simulink model "BaseEngineController_LS"  (Simulink 7.7)
settings: Solver=FixedStepDiscrete  StartTime=0.0  StopTime=10.0  RelTol=1e-3
PreLoadFcn:
  | try, eval([bdroot '_setup']); catch, eval('model_setup', ''); end
InitFcn:
  | try, eval([bdroot '_setup']); catch, eval('model_setup', ''); end
undefined symbols (not defined in the file): ECU555, High, motohawk_build_version, motohawk_trunc_name, motohawk_vardec_config_group, motohawk_vardec_path, True
libraries: MotoHawk_lib x1418, motohawk_control_primitives_lib x183, motohawk_engine_lib x32, simulink x21, motohawk_annotations_lib x9, AutoDoc_lib x8, simulink_extras x4, motohawk_ccp_examples_lib x1, motohawk_control_primitives_motoshare_lib x1
(part 15 of 27)

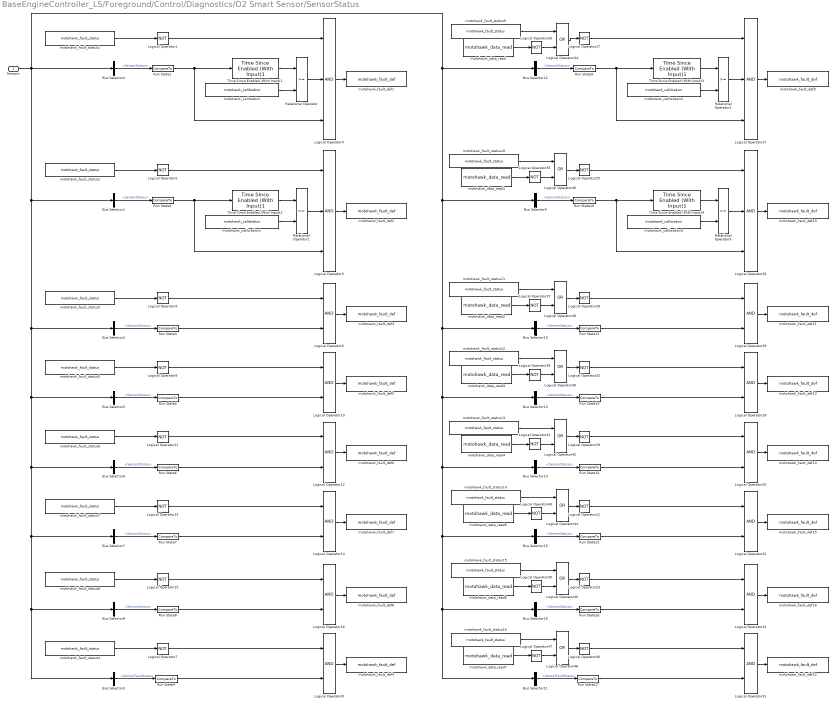
== system BaseEngineController_LS/Foreground/Control/Diagnostics/O2 Smart Sensor/SensorStatus ==
  Sensors : Inport
  Bus Selector{1..2,4..8} (7 alike) : BusSelector  OutputSignals=Raw.CAN.O2_BUS.BANK1.SensorStatus
  Bus Selector{9..10,12..16} (7 alike) : BusSelector  OutputSignals=Raw.CAN.O2_BUS.BANK2.SensorStatus
  Bus Selector11 : BusSelector  OutputSignals=Raw.CAN.O2_BUS.BANK2.SensorFaultState
  Bus Selector3 : BusSelector  OutputSignals=Raw.CAN.O2_BUS.BANK1.SensorFaultState
  Logical Operator{1..2,5,7,9,11,13,15,17,19,21,23,25,28,30,32..33,35,37,39,41,43,45,47} (24 alike) : Logic  Operator=NOT  Inputs=3  AllPortsSameDT=off  OutDataTypeStr=boolean
  Logical Operator{6,8,10,12,14,16,18,20,22,24,29,31} (12 alike) : Logic  AllPortsSameDT=off  OutDataTypeStr=boolean
  Logical Operator{3..4,26..27} (4 alike) : Logic  Inputs=3  AllPortsSameDT=off  OutDataTypeStr=boolean
  Logical Operator{34,36,38,40,42,44,46,48} (8 alike) : Logic  Operator=OR  AllPortsSameDT=off  OutDataTypeStr=boolean
  Relational Operator{,1..3} (4 alike) : RelationalOperator  OutDataTypeStr=boolean
  Run State1 : motohawk_control_primitives_lib/CompareTo  SystemSampleTime=-1  op===  val=0
  Run State{2,4,10,12} (4 alike) : motohawk_control_primitives_lib/CompareTo  SystemSampleTime=-1  op===  val=1
  Run State11 : motohawk_control_primitives_lib/CompareTo  SystemSampleTime=-1  op===  val=7
  Run State13 : motohawk_control_primitives_lib/CompareTo  SystemSampleTime=-1  op===  val=8
  Run State14 : motohawk_control_primitives_lib/CompareTo  SystemSampleTime=-1  op===  val=9
  Run State15 : motohawk_control_primitives_lib/CompareTo  SystemSampleTime=-1  op===  val=10
  Run State16 : motohawk_control_primitives_lib/CompareTo  SystemSampleTime=-1  op===  val=20
  Run State3 : motohawk_control_primitives_lib/CompareTo  SystemSampleTime=-1  op===  val=7
  Run State5 : motohawk_control_primitives_lib/CompareTo  SystemSampleTime=-1  op===  val=8
  Run State6 : motohawk_control_primitives_lib/CompareTo  SystemSampleTime=-1  op===  val=9
  Run State7 : motohawk_control_primitives_lib/CompareTo  SystemSampleTime=-1  op===  val=10
  Run State8 : motohawk_control_primitives_lib/CompareTo  SystemSampleTime=-1  op===  val=20
  Run State9 : motohawk_control_primitives_lib/CompareTo  SystemSampleTime=-1  op===  val=0
  Time Since Enabled (With Input)1 : motohawk_control_primitives_lib/Time Since Enabled (With Input)1  SystemSampleTime=-1  nam='Lam1ResetTime'  samp_time=-1  init=0  upperlim=16000
  Time Since Enabled (With Input)2 : motohawk_control_primitives_lib/Time Since Enabled (With Input)1  SystemSampleTime=-1  nam='Lam1WarmupTime'  samp_time=-1  init=0  upperlim=16000
  Time Since Enabled (With Input)3 : motohawk_control_primitives_lib/Time Since Enabled (With Input)1  SystemSampleTime=-1  nam='Lam2ResetTime'  samp_time=-1  init=0  upperlim=16000
  Time Since Enabled (With Input)4 : motohawk_control_primitives_lib/Time Since Enabled (With Input)1  SystemSampleTime=-1  nam='Lam2WarmupTime'  samp_time=-1  init=0  upperlim=16000
  motohawk_calibration : MotoHawk_lib/Calibration & Probing Blocks/motohawk_calibration  nam='O2Diag_Lam1_StuckInResetThresh'  val=30  storage=Calibration  show_more=off  name_source=Use Parameter  data_type=Inherit from 'Default Value'  read_level=1  write_level=1  ovr_cals=on  view_as=Number  enum_struct={'Disabled', 'Enabled'}  vector_style=Wide Row  use_help_units=off  help=''  units=''  use_header_enum=off  row_header_enum={}  col_header_enum={}  use_min_max=off  min_val=-inf  max_val=inf  use_precision=off  precision=''  gain=1  offset=0  exp=1  use_mototune_group=off  mototune_group=motohawk_vardec_path(gcb)
  motohawk_calibration1 : MotoHawk_lib/Calibration & Probing Blocks/motohawk_calibration  nam='O2Diag_Lam1_StuckInWarmup'  val=30  storage=Calibration  show_more=off  name_source=Use Parameter  data_type=Inherit from 'Default Value'  read_level=1  write_level=1  ovr_cals=on  view_as=Number  enum_struct={'Disabled', 'Enabled'}  vector_style=Wide Row  use_help_units=off  help=''  units=''  use_header_enum=off  row_header_enum={}  col_header_enum={}  use_min_max=off  min_val=-inf  max_val=inf  use_precision=off  precision=''  gain=1  offset=0  exp=1  use_mototune_group=off  mototune_group=motohawk_vardec_path(gcb)
  motohawk_calibration2 : MotoHawk_lib/Calibration & Probing Blocks/motohawk_calibration  nam='O2Diag_Lam21_StuckInResetThresh'  val=30  storage=Calibration  show_more=off  name_source=Use Parameter  data_type=Inherit from 'Default Value'  read_level=1  write_level=1  ovr_cals=on  view_as=Number  enum_struct={'Disabled', 'Enabled'}  vector_style=Wide Row  use_help_units=off  help=''  units=''  use_header_enum=off  row_header_enum={}  col_header_enum={}  use_min_max=off  min_val=-inf  max_val=inf  use_precision=off  precision=''  gain=1  offset=0  exp=1  use_mototune_group=off  mototune_group=motohawk_vardec_path(gcb)
  motohawk_calibration3 : MotoHawk_lib/Calibration & Probing Blocks/motohawk_calibration  nam='O2Diag_Lam2_StuckInWarmup'  val=30  storage=Calibration  show_more=off  name_source=Use Parameter  data_type=Inherit from 'Default Value'  read_level=1  write_level=1  ovr_cals=on  view_as=Number  enum_struct={'Disabled', 'Enabled'}  vector_style=Wide Row  use_help_units=off  help=''  units=''  use_header_enum=off  row_header_enum={}  col_header_enum={}  use_min_max=off  min_val=-inf  max_val=inf  use_precision=off  precision=''  gain=1  offset=0  exp=1  use_mototune_group=off  mototune_group=motohawk_vardec_path(gcb)
  motohawk_data_read{,1..7} (8 alike) : MotoHawk_lib/Data Storage Blocks/motohawk_data_read  source=Lookup By Name  structure=Scalar  operation=Read scalar from location by index  sz_vec=4  sz_row=2  sz_col=3  typ=boolean  nam='BankB_Enbl'  checkNull=on  struct_inst_name='MyData'  struct_nam='MyStruct'
  motohawk_fault_def1 : MotoHawk_lib/Fault Management Blocks/motohawk_fault_def  nam='Lambda1StuckInReset_Fault'  mode=Enabled  id=[]  x=25  y=50  input_suspected=on  indeterminate=off  increment_xy=on  downsample_count=1  ovr_cals=on  ovr_actions=on  show_actions=on  action1_name=''  action1_cond=(None)  action2_name=''  action2_cond=(None)  action3_name=''  action3_cond=(None)  action4_name=''  action4_cond=(None)
  motohawk_fault_def10 : MotoHawk_lib/Fault Management Blocks/motohawk_fault_def  nam='Lambda2StuckInWarmup_Fault'  mode=Enabled  id=[]  x=25  y=50  input_suspected=on  indeterminate=off  increment_xy=on  downsample_count=1  ovr_cals=on  ovr_actions=on  show_actions=on  action1_name=''  action1_cond=(None)  action2_name=''  action2_cond=(None)  action3_name=''  action3_cond=(None)  action4_name=''  action4_cond=(None)
  motohawk_fault_def11 : MotoHawk_lib/Fault Management Blocks/motohawk_fault_def  nam='Lambda2Overheat_Fault'  mode=Enabled  id=[]  x=25  y=50  input_suspected=on  indeterminate=off  increment_xy=on  downsample_count=1  ovr_cals=on  ovr_actions=on  show_actions=on  action1_name=''  action1_cond=(None)  action2_name=''  action2_cond=(None)  action3_name=''  action3_cond=(None)  action4_name=''  action4_cond=(None)
  motohawk_fault_def12 : MotoHawk_lib/Fault Management Blocks/motohawk_fault_def  nam='Lambda2Fault_Fault'  mode=Enabled  id=[]  x=25  y=50  input_suspected=on  indeterminate=off  increment_xy=on  downsample_count=1  ovr_cals=on  ovr_actions=on  show_actions=on  action1_name=''  action1_cond=(None)  action2_name=''  action2_cond=(None)  action3_name=''  action3_cond=(None)  action4_name=''  action4_cond=(None)
  motohawk_fault_def13 : MotoHawk_lib/Fault Management Blocks/motohawk_fault_def  nam='Lambda2Overcool_Fault'  mode=Enabled  id=[]  x=25  y=50  input_suspected=on  indeterminate=off  increment_xy=on  downsample_count=1  ovr_cals=on  ovr_actions=on  show_actions=on  action1_name=''  action1_cond=(None)  action2_name=''  action2_cond=(None)  action3_name=''  action3_cond=(None)  action4_name=''  action4_cond=(None)
  motohawk_fault_def14 : MotoHawk_lib/Fault Management Blocks/motohawk_fault_def  nam='Lambda2HtrShort_Fault'  mode=Enabled  id=[]  x=25  y=50  input_suspected=on  indeterminate=off  increment_xy=on  downsample_count=1  ovr_cals=on  ovr_actions=on  show_actions=on  action1_name=''  action1_cond=(None)  action2_name=''  action2_cond=(None)  action3_name=''  action3_cond=(None)  action4_name=''  action4_cond=(None)
  motohawk_fault_def15 : MotoHawk_lib/Fault Management Blocks/motohawk_fault_def  nam='Lambda2HtrOpen_Fault'  mode=Enabled  id=[]  x=25  y=50  input_suspected=on  indeterminate=off  increment_xy=on  downsample_count=1  ovr_cals=on  ovr_actions=on  show_actions=on  action1_name=''  action1_cond=(None)  action2_name=''  action2_cond=(None)  action3_name=''  action3_cond=(None)  action4_name=''  action4_cond=(None)
  motohawk_fault_def16 : MotoHawk_lib/Fault Management Blocks/motohawk_fault_def  nam='Lambda2Error_Fault'  mode=Enabled  id=[]  x=25  y=50  input_suspected=on  indeterminate=off  increment_xy=on  downsample_count=1  ovr_cals=on  ovr_actions=on  show_actions=on  action1_name=''  action1_cond=(None)  action2_name=''  action2_cond=(None)  action3_name=''  action3_cond=(None)  action4_name=''  action4_cond=(None)
  motohawk_fault_def2 : MotoHawk_lib/Fault Management Blocks/motohawk_fault_def  nam='Lambda1StuckInWarmup_Fault'  mode=Enabled  id=[]  x=25  y=50  input_suspected=on  indeterminate=off  increment_xy=on  downsample_count=1  ovr_cals=on  ovr_actions=on  show_actions=on  action1_name=''  action1_cond=(None)  action2_name=''  action2_cond=(None)  action3_name=''  action3_cond=(None)  action4_name=''  action4_cond=(None)
  motohawk_fault_def3 : MotoHawk_lib/Fault Management Blocks/motohawk_fault_def  nam='Lambda1Overheat_Fault'  mode=Enabled  id=[]  x=25  y=50  input_suspected=on  indeterminate=off  increment_xy=on  downsample_count=1  ovr_cals=on  ovr_actions=on  show_actions=on  action1_name=''  action1_cond=(None)  action2_name=''  action2_cond=(None)  action3_name=''  action3_cond=(None)  action4_name=''  action4_cond=(None)
  motohawk_fault_def4 : MotoHawk_lib/Fault Management Blocks/motohawk_fault_def  nam='Lambda1Fault_Fault'  mode=Enabled  id=[]  x=25  y=50  input_suspected=on  indeterminate=off  increment_xy=on  downsample_count=1  ovr_cals=on  ovr_actions=on  show_actions=on  action1_name=''  action1_cond=(None)  action2_name=''  action2_cond=(None)  action3_name=''  action3_cond=(None)  action4_name=''  action4_cond=(None)
  motohawk_fault_def5 : MotoHawk_lib/Fault Management Blocks/motohawk_fault_def  nam='Lambda1Overcool_Fault'  mode=Enabled  id=[]  x=25  y=50  input_suspected=on  indeterminate=off  increment_xy=on  downsample_count=1  ovr_cals=on  ovr_actions=on  show_actions=on  action1_name=''  action1_cond=(None)  action2_name=''  action2_cond=(None)  action3_name=''  action3_cond=(None)  action4_name=''  action4_cond=(None)
  motohawk_fault_def6 : MotoHawk_lib/Fault Management Blocks/motohawk_fault_def  nam='Lambda1HtrShort_Fault'  mode=Enabled  id=[]  x=25  y=50  input_suspected=on  indeterminate=off  increment_xy=on  downsample_count=1  ovr_cals=on  ovr_actions=on  show_actions=on  action1_name=''  action1_cond=(None)  action2_name=''  action2_cond=(None)  action3_name=''  action3_cond=(None)  action4_name=''  action4_cond=(None)
  motohawk_fault_def7 : MotoHawk_lib/Fault Management Blocks/motohawk_fault_def  nam='Lambda1HtrOpen_Fault'  mode=Enabled  id=[]  x=25  y=50  input_suspected=on  indeterminate=off  increment_xy=on  downsample_count=1  ovr_cals=on  ovr_actions=on  show_actions=on  action1_name=''  action1_cond=(None)  action2_name=''  action2_cond=(None)  action3_name=''  action3_cond=(None)  action4_name=''  action4_cond=(None)
  motohawk_fault_def8 : MotoHawk_lib/Fault Management Blocks/motohawk_fault_def  nam='Lambda1Error_Fault'  mode=Enabled  id=[]  x=25  y=50  input_suspected=on  indeterminate=off  increment_xy=on  downsample_count=1  ovr_cals=on  ovr_actions=on  show_actions=on  action1_name=''  action1_cond=(None)  action2_name=''  action2_cond=(None)  action3_name=''  action3_cond=(None)  action4_name=''  action4_cond=(None)
  motohawk_fault_def9 : MotoHawk_lib/Fault Management Blocks/motohawk_fault_def  nam='Lambda2StuckInReset_Fault'  mode=Enabled  id=[]  x=25  y=50  input_suspected=on  indeterminate=off  increment_xy=on  downsample_count=1  ovr_cals=on  ovr_actions=on  show_actions=on  action1_name=''  action1_cond=(None)  action2_name=''  action2_cond=(None)  action3_name=''  action3_cond=(None)  action4_name=''  action4_cond=(None)
  motohawk_fault_status{1..8} (8 alike) : MotoHawk_lib/Fault Management Blocks/motohawk_fault_status  source=Lookup By Name  nam='Lambda_1_Timeout'  status=Active
  motohawk_fault_status{9..16} (8 alike) : MotoHawk_lib/Fault Management Blocks/motohawk_fault_status  source=Lookup By Name  nam='Lambda_2_Timeout'  status=Active
  wires:
  Logical Operator4/1 -> motohawk_fault_def1/1
  motohawk_fault_status1/1 -> Logical Operator1/1
  Sensors/1 -> Bus Selector4/1, Bus Selector1/1, Bus Selector2/1, Bus Selector5/1, Bus Selector6/1, Bus Selector7/1, Bus Selector8/1, Bus Selector3/1, Bus Selector12/1, Bus Selector9/1, Bus Selector10/1, Bus Selector13/1, Bus Selector14/1, Bus Selector15/1, Bus Selector11/1, Bus Selector16/1
  Logical Operator1/1 -> Logical Operator4/1
  Bus Selector4/1 -> Run State1/1  "<SensorStatus>"
  Time Since Enabled (With Input)1/1 -> Relational Operator/1
  motohawk_calibration/1 -> Relational Operator/2
  Run State1/1 -> Time Since Enabled (With Input)1/1, Logical Operator4/3
  Relational Operator/1 -> Logical Operator4/2
  Logical Operator3/1 -> motohawk_fault_def2/1
  motohawk_fault_status2/1 -> Logical Operator2/1
  Logical Operator2/1 -> Logical Operator3/1
  Bus Selector1/1 -> Run State2/1  "<SensorStatus>"
  Time Since Enabled (With Input)2/1 -> Relational Operator1/1
  motohawk_calibration1/1 -> Relational Operator1/2
  Run State2/1 -> Time Since Enabled (With Input)2/1, Logical Operator3/3
  Relational Operator1/1 -> Logical Operator3/2
  Logical Operator6/1 -> motohawk_fault_def3/1
  motohawk_fault_status3/1 -> Logical Operator5/1
  Logical Operator5/1 -> Logical Operator6/1
  Bus Selector2/1 -> Run State3/1  "<SensorStatus>"
  Run State3/1 -> Logical Operator6/2
  Logical Operator8/1 -> motohawk_fault_def4/1
  motohawk_fault_status4/1 -> Logical Operator7/1
  Logical Operator7/1 -> Logical Operator8/1
  Bus Selector3/1 -> Run State4/1  "<SensorFaultState>"
  Run State4/1 -> Logical Operator8/2
  Logical Operator10/1 -> motohawk_fault_def5/1
  motohawk_fault_status5/1 -> Logical Operator9/1
  Logical Operator9/1 -> Logical Operator10/1
  Bus Selector5/1 -> Run State5/1  "<SensorStatus>"
  Run State5/1 -> Logical Operator10/2
  Logical Operator12/1 -> motohawk_fault_def6/1
  motohawk_fault_status6/1 -> Logical Operator11/1
  Logical Operator11/1 -> Logical Operator12/1
  Bus Selector6/1 -> Run State6/1  "<SensorStatus>"
  Run State6/1 -> Logical Operator12/2
  Logical Operator14/1 -> motohawk_fault_def7/1
  motohawk_fault_status7/1 -> Logical Operator13/1
  Logical Operator13/1 -> Logical Operator14/1
  Bus Selector7/1 -> Run State7/1  "<SensorStatus>"
  Run State7/1 -> Logical Operator14/2
  Logical Operator16/1 -> motohawk_fault_def8/1
  motohawk_fault_status8/1 -> Logical Operator15/1
  Logical Operator15/1 -> Logical Operator16/1
  Bus Selector8/1 -> Run State8/1  "<SensorStatus>"
  Run State8/1 -> Logical Operator16/2
  Logical Operator27/1 -> motohawk_fault_def9/1
  Logical Operator17/1 -> Logical Operator27/1
  Bus Selector12/1 -> Run State9/1  "<SensorStatus>"
  Time Since Enabled (With Input)3/1 -> Relational Operator2/1
  motohawk_calibration2/1 -> Relational Operator2/2
  Run State9/1 -> Time Since Enabled (With Input)3/1, Logical Operator27/3
  Relational Operator2/1 -> Logical Operator27/2
  Logical Operator26/1 -> motohawk_fault_def10/1
  Logical Operator25/1 -> Logical Operator26/1
  Bus Selector9/1 -> Run State10/1  "<SensorStatus>"
  Time Since Enabled (With Input)4/1 -> Relational Operator3/1
  motohawk_calibration3/1 -> Relational Operator3/2
  Run State10/1 -> Time Since Enabled (With Input)4/1, Logical Operator26/3
  Relational Operator3/1 -> Logical Operator26/2
  Logical Operator29/1 -> motohawk_fault_def11/1
  Logical Operator28/1 -> Logical Operator29/1
  Bus Selector10/1 -> Run State11/1  "<SensorStatus>"
  Run State11/1 -> Logical Operator29/2
  Logical Operator31/1 -> motohawk_fault_def12/1
  Logical Operator30/1 -> Logical Operator31/1
  Bus Selector11/1 -> Run State12/1  "<SensorFaultState>"
  Run State12/1 -> Logical Operator31/2
  Logical Operator18/1 -> motohawk_fault_def13/1
  Logical Operator32/1 -> Logical Operator18/1
  Bus Selector13/1 -> Run State13/1  "<SensorStatus>"
  Run State13/1 -> Logical Operator18/2
  Logical Operator20/1 -> motohawk_fault_def14/1
  Logical Operator19/1 -> Logical Operator20/1
  Bus Selector14/1 -> Run State14/1  "<SensorStatus>"
  Run State14/1 -> Logical Operator20/2
  Logical Operator22/1 -> motohawk_fault_def15/1
  Logical Operator21/1 -> Logical Operator22/1
  Bus Selector15/1 -> Run State15/1  "<SensorStatus>"
  Run State15/1 -> Logical Operator22/2
  Logical Operator24/1 -> motohawk_fault_def16/1
  Logical Operator23/1 -> Logical Operator24/1
  Bus Selector16/1 -> Run State16/1  "<SensorStatus>"
  Run State16/1 -> Logical Operator24/2
  motohawk_data_read/1 -> Logical Operator33/1
  Logical Operator33/1 -> Logical Operator34/2
  motohawk_fault_status9/1 -> Logical Operator34/1
  Logical Operator34/1 -> Logical Operator17/1
  motohawk_data_read1/1 -> Logical Operator35/1
  Logical Operator35/1 -> Logical Operator36/2
  motohawk_fault_status10/1 -> Logical Operator36/1
  Logical Operator36/1 -> Logical Operator25/1
  motohawk_data_read2/1 -> Logical Operator37/1
  Logical Operator37/1 -> Logical Operator38/2
  motohawk_fault_status11/1 -> Logical Operator38/1
  Logical Operator38/1 -> Logical Operator28/1
  motohawk_data_read3/1 -> Logical Operator39/1
  Logical Operator39/1 -> Logical Operator40/2
  motohawk_fault_status12/1 -> Logical Operator40/1
  Logical Operator40/1 -> Logical Operator32/1
  motohawk_data_read4/1 -> Logical Operator41/1
  Logical Operator41/1 -> Logical Operator42/2
  motohawk_fault_status13/1 -> Logical Operator42/1
  Logical Operator42/1 -> Logical Operator19/1
  motohawk_data_read5/1 -> Logical Operator43/1
  Logical Operator43/1 -> Logical Operator44/2
  motohawk_fault_status14/1 -> Logical Operator44/1
  Logical Operator44/1 -> Logical Operator21/1
  motohawk_data_read6/1 -> Logical Operator45/1
  Logical Operator45/1 -> Logical Operator46/2
  motohawk_fault_status15/1 -> Logical Operator46/1
  Logical Operator46/1 -> Logical Operator23/1
  motohawk_data_read7/1 -> Logical Operator47/1
  Logical Operator47/1 -> Logical Operator48/2
  motohawk_fault_status16/1 -> Logical Operator48/1
  Logical Operator48/1 -> Logical Operator30/1

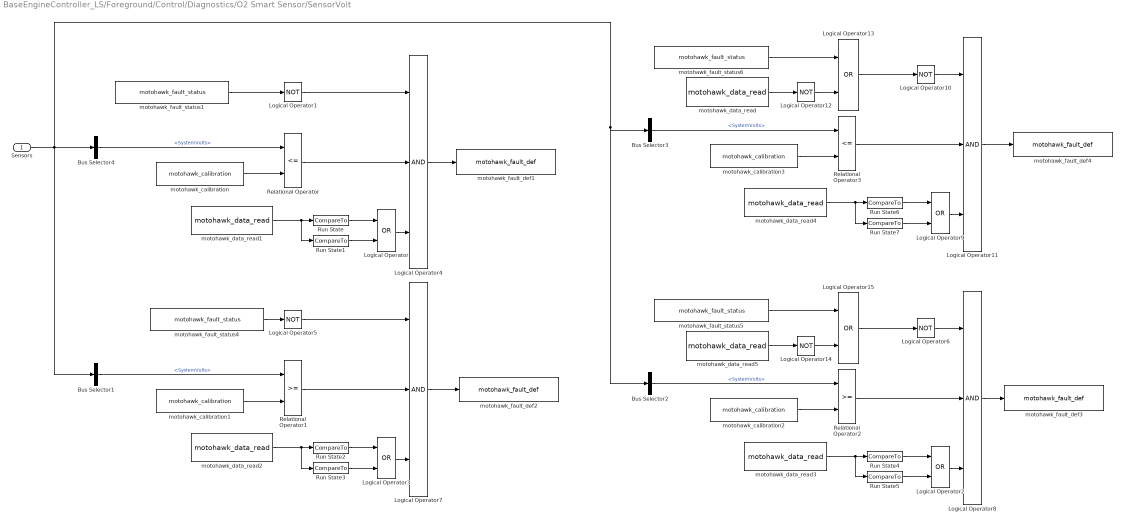
== system BaseEngineController_LS/Foreground/Control/Diagnostics/O2 Smart Sensor/SensorVolt ==
  Sensors : Inport
  Bus Selector1 : BusSelector  OutputSignals=Raw.CAN.O2_BUS.BANK1.SystemVolts
  Bus Selector2 : BusSelector  OutputSignals=Raw.CAN.O2_BUS.BANK2.SystemVolts
  Bus Selector3 : BusSelector  OutputSignals=Raw.CAN.O2_BUS.BANK2.SystemVolts
  Bus Selector4 : BusSelector  OutputSignals=Raw.CAN.O2_BUS.BANK1.SystemVolts
  Logical Operator{,2..3,9,13,15} (6 alike) : Logic  Operator=OR  AllPortsSameDT=off  OutDataTypeStr=boolean
  Logical Operator{1,5..6,10,12,14} (6 alike) : Logic  Operator=NOT  Inputs=3  AllPortsSameDT=off  OutDataTypeStr=boolean
  Logical Operator{4,7..8,11} (4 alike) : Logic  Inputs=3  AllPortsSameDT=off  OutDataTypeStr=boolean
  Relational Operator : RelationalOperator  Operator=<=  OutDataTypeStr=boolean
  Relational Operator1 : RelationalOperator  OutDataTypeStr=boolean
  Relational Operator2 : RelationalOperator  OutDataTypeStr=boolean
  Relational Operator3 : RelationalOperator  Operator=<=  OutDataTypeStr=boolean
  Run State{,2,4,6} (4 alike) : motohawk_control_primitives_lib/CompareTo  SystemSampleTime=-1  op===  val=3
  Run State{1,3,5,7} (4 alike) : motohawk_control_primitives_lib/CompareTo  SystemSampleTime=-1  op===  val=2
  motohawk_calibration : MotoHawk_lib/Calibration & Probing Blocks/motohawk_calibration  nam='Lambda1_VoltLowThresh'  val=10  storage=Calibration  show_more=off  name_source=Use Parameter  data_type=Inherit from 'Default Value'  read_level=1  write_level=1  ovr_cals=on  view_as=Number  enum_struct={'Disabled', 'Enabled'}  vector_style=Wide Row  use_help_units=off  help=''  units=''  use_header_enum=off  row_header_enum={}  col_header_enum={}  use_min_max=off  min_val=-inf  max_val=inf  use_precision=off  precision=''  gain=1  offset=0  exp=1  use_mototune_group=off  mototune_group=motohawk_vardec_path(gcb)
  motohawk_calibration1 : MotoHawk_lib/Calibration & Probing Blocks/motohawk_calibration  nam='Lambda1_VoltHighThresh'  val=15  storage=Calibration  show_more=off  name_source=Use Parameter  data_type=Inherit from 'Default Value'  read_level=1  write_level=1  ovr_cals=on  view_as=Number  enum_struct={'Disabled', 'Enabled'}  vector_style=Wide Row  use_help_units=off  help=''  units=''  use_header_enum=off  row_header_enum={}  col_header_enum={}  use_min_max=off  min_val=-inf  max_val=inf  use_precision=off  precision=''  gain=1  offset=0  exp=1  use_mototune_group=off  mototune_group=motohawk_vardec_path(gcb)
  motohawk_calibration2 : MotoHawk_lib/Calibration & Probing Blocks/motohawk_calibration  nam='Lambda2_VoltHighThresh'  val=15  storage=Calibration  show_more=off  name_source=Use Parameter  data_type=Inherit from 'Default Value'  read_level=1  write_level=1  ovr_cals=on  view_as=Number  enum_struct={'Disabled', 'Enabled'}  vector_style=Wide Row  use_help_units=off  help=''  units=''  use_header_enum=off  row_header_enum={}  col_header_enum={}  use_min_max=off  min_val=-inf  max_val=inf  use_precision=off  precision=''  gain=1  offset=0  exp=1  use_mototune_group=off  mototune_group=motohawk_vardec_path(gcb)
  motohawk_calibration3 : MotoHawk_lib/Calibration & Probing Blocks/motohawk_calibration  nam='Lambda2_VoltLowThresh'  val=10  storage=Calibration  show_more=off  name_source=Use Parameter  data_type=Inherit from 'Default Value'  read_level=1  write_level=1  ovr_cals=on  view_as=Number  enum_struct={'Disabled', 'Enabled'}  vector_style=Wide Row  use_help_units=off  help=''  units=''  use_header_enum=off  row_header_enum={}  col_header_enum={}  use_min_max=off  min_val=-inf  max_val=inf  use_precision=off  precision=''  gain=1  offset=0  exp=1  use_mototune_group=off  mototune_group=motohawk_vardec_path(gcb)
  motohawk_data_read : MotoHawk_lib/Data Storage Blocks/motohawk_data_read  source=Lookup By Name  structure=Scalar  operation=Read scalar from location by index  sz_vec=4  sz_row=2  sz_col=3  typ=boolean  nam='BankB_Enbl'  checkNull=on  struct_inst_name='MyData'  struct_nam='MyStruct'
  motohawk_data_read{1..4} (4 alike) : MotoHawk_lib/Data Storage Blocks/motohawk_data_read  source=Lookup By Name  structure=Scalar  operation=Read entire data structure at once  sz_vec=4  sz_row=2  sz_col=3  typ=uint8  nam='EngineState'  checkNull=on  struct_inst_name='Struct1'  struct_nam='MyStruct'
  motohawk_data_read5 : MotoHawk_lib/Data Storage Blocks/motohawk_data_read  source=Lookup By Name  structure=Scalar  operation=Read scalar from location by index  sz_vec=4  sz_row=2  sz_col=3  typ=boolean  nam='BankB_Enbl'  checkNull=on  struct_inst_name='MyData'  struct_nam='MyStruct'
  motohawk_fault_def1 : MotoHawk_lib/Fault Management Blocks/motohawk_fault_def  nam='Lambda1VoltLow_Fault'  mode=Enabled  id=[]  x=25  y=50  input_suspected=on  indeterminate=off  increment_xy=on  downsample_count=1  ovr_cals=on  ovr_actions=on  show_actions=on  action1_name=''  action1_cond=(None)  action2_name=''  action2_cond=(None)  action3_name=''  action3_cond=(None)  action4_name=''  action4_cond=(None)
  motohawk_fault_def2 : MotoHawk_lib/Fault Management Blocks/motohawk_fault_def  nam='Lambda1VoltHigh_Fault'  mode=Enabled  id=[]  x=25  y=50  input_suspected=on  indeterminate=off  increment_xy=on  downsample_count=1  ovr_cals=on  ovr_actions=on  show_actions=on  action1_name=''  action1_cond=(None)  action2_name=''  action2_cond=(None)  action3_name=''  action3_cond=(None)  action4_name=''  action4_cond=(None)
  motohawk_fault_def3 : MotoHawk_lib/Fault Management Blocks/motohawk_fault_def  nam='Lambda2VoltHigh_Fault'  mode=Enabled  id=[]  x=25  y=50  input_suspected=on  indeterminate=off  increment_xy=on  downsample_count=1  ovr_cals=on  ovr_actions=on  show_actions=on  action1_name=''  action1_cond=(None)  action2_name=''  action2_cond=(None)  action3_name=''  action3_cond=(None)  action4_name=''  action4_cond=(None)
  motohawk_fault_def4 : MotoHawk_lib/Fault Management Blocks/motohawk_fault_def  nam='Lambda2VoltLow_Fault'  mode=Enabled  id=[]  x=25  y=50  input_suspected=on  indeterminate=off  increment_xy=on  downsample_count=1  ovr_cals=on  ovr_actions=on  show_actions=on  action1_name=''  action1_cond=(None)  action2_name=''  action2_cond=(None)  action3_name=''  action3_cond=(None)  action4_name=''  action4_cond=(None)
  motohawk_fault_status1 : MotoHawk_lib/Fault Management Blocks/motohawk_fault_status  source=Lookup By Name  nam='Lambda_1_Timeout'  status=Active
  motohawk_fault_status4 : MotoHawk_lib/Fault Management Blocks/motohawk_fault_status  source=Lookup By Name  nam='Lambda_1_Timeout'  status=Active
  motohawk_fault_status5 : MotoHawk_lib/Fault Management Blocks/motohawk_fault_status  source=Lookup By Name  nam='Lambda_2_Timeout'  status=Active
  motohawk_fault_status6 : MotoHawk_lib/Fault Management Blocks/motohawk_fault_status  source=Lookup By Name  nam='Lambda_2_Timeout'  status=Active
  wires:
  Sensors/1 -> Bus Selector4/1, Bus Selector1/1, Bus Selector2/1, Bus Selector3/1
  Logical Operator4/1 -> motohawk_fault_def1/1
  Logical Operator1/1 -> Logical Operator4/1
  motohawk_data_read1/1 -> Run State/1, Run State1/1
  Run State1/1 -> Logical Operator/2
  Run State/1 -> Logical Operator/1
  Logical Operator/1 -> Logical Operator4/3
  Bus Selector4/1 -> Relational Operator/1  "<SystemVolts>"
  Relational Operator/1 -> Logical Operator4/2
  motohawk_calibration/1 -> Relational Operator/2
  motohawk_fault_status1/1 -> Logical Operator1/1
  Logical Operator7/1 -> motohawk_fault_def2/1
  Logical Operator5/1 -> Logical Operator7/1
  motohawk_data_read2/1 -> Run State2/1, Run State3/1
  Run State3/1 -> Logical Operator3/2
  Run State2/1 -> Logical Operator3/1
  Logical Operator3/1 -> Logical Operator7/3
  Bus Selector1/1 -> Relational Operator1/1  "<SystemVolts>"
  Relational Operator1/1 -> Logical Operator7/2
  motohawk_calibration1/1 -> Relational Operator1/2
  motohawk_fault_status4/1 -> Logical Operator5/1
  Logical Operator8/1 -> motohawk_fault_def3/1
  motohawk_data_read3/1 -> Run State4/1, Run State5/1
  Run State5/1 -> Logical Operator2/2
  Run State4/1 -> Logical Operator2/1
  Logical Operator2/1 -> Logical Operator8/3
  Bus Selector2/1 -> Relational Operator2/1  "<SystemVolts>"
  Relational Operator2/1 -> Logical Operator8/2
  motohawk_calibration2/1 -> Relational Operator2/2
  Logical Operator11/1 -> motohawk_fault_def4/1
  Logical Operator10/1 -> Logical Operator11/1
  motohawk_data_read4/1 -> Run State6/1, Run State7/1
  Run State7/1 -> Logical Operator9/2
  Run State6/1 -> Logical Operator9/1
  Logical Operator9/1 -> Logical Operator11/3
  Bus Selector3/1 -> Relational Operator3/1  "<SystemVolts>"
  Relational Operator3/1 -> Logical Operator11/2
  motohawk_calibration3/1 -> Relational Operator3/2
  motohawk_data_read/1 -> Logical Operator12/1
  Logical Operator12/1 -> Logical Operator13/2
  motohawk_fault_status6/1 -> Logical Operator13/1
  Logical Operator13/1 -> Logical Operator10/1
  motohawk_data_read5/1 -> Logical Operator14/1
  Logical Operator14/1 -> Logical Operator15/2
  motohawk_fault_status5/1 -> Logical Operator15/1
  Logical Operator15/1 -> Logical Operator6/1
  Logical Operator6/1 -> Logical Operator8/1

== system BaseEngineController_LS/Foreground/Control/Diagnostics/Overspeed Protection/BaseRevLimit ==
  RPM : Inport
  Hysterisis : motohawk_control_primitives_lib/Hysterisis  SystemSampleTime=-1
  Hysterisis1 : motohawk_control_primitives_lib/Hysterisis  SystemSampleTime=-1
  Hysterisis2 : motohawk_control_primitives_lib/Hysterisis  SystemSampleTime=-1
  Logical Operator3 : Logic
  Logical Operator4 : Logic  Operator=NOT
  Logical Operator5 : Logic
  Logical Operator6 : Logic  Operator=NOT
  Overspeed : RelationalOperator  Operator=>  ZeroCross=off  InputSameDT=on
  Overspeed1 : RelationalOperator  Operator=>  ZeroCross=off  InputSameDT=on
  Overspeed2 : RelationalOperator  Operator=>  ZeroCross=off  InputSameDT=on
  Sum1 : Sum  Inputs=+-  SaturateOnIntegerOverflow=on
  Sum2 : Sum  Inputs=+-  SaturateOnIntegerOverflow=on
  Sum3 : Sum  SaturateOnIntegerOverflow=on
  Sum4 : Sum  Inputs=+-  SaturateOnIntegerOverflow=on
  Sum5 : Sum  SaturateOnIntegerOverflow=on
  motohawk_calibration : MotoHawk_lib/Calibration & Probing Blocks/motohawk_calibration  nam='BaseRevLimit'  val=4200  storage=Calibration  show_more=on  name_source=Use Parameter  data_type=int16  read_level=1  write_level=1  ovr_cals=on  view_as=Number  enum_struct={'Disabled', 'Enabled'}  vector_style=Wide Row  use_help_units=on  help='Maximum RPM allowed, before any action is taken'  units='RPM'  use_header_enum=off  row_header_enum={}  col_header_enum={}  use_min_max=on  min_val=0  max_val=inf  use_precision=off  precision=''  gain=1  offset=0  exp=1  use_mototune_group=on  mototune_group=motohawk_vardec_path(gcb)
  motohawk_calibration1 : MotoHawk_lib/Calibration & Probing Blocks/motohawk_calibration  nam='RevLimitHyst'  val=20  storage=Calibration  show_more=on  name_source=Use Parameter  data_type=int16  read_level=1  write_level=1  ovr_cals=on  view_as=Number  enum_struct={'Disabled', 'Enabled'}  vector_style=Wide Row  use_help_units=on  help='Hysteresis applied to MaxRPM once rev limit threshold is satisfied'  units='RPM'  use_header_enum=off  row_header_enum={}  col_header_enum={}  use_min_max=on  min_val=0  max_val=12000  use_precision=off  precision=''  gain=1  offset=0  exp=1  use_mototune_group=on  mototune_group=motohawk_vardec_path(gcb)
  motohawk_calibration2 : MotoHawk_lib/Calibration & Probing Blocks/motohawk_calibration  nam='MediumRevOffset'  val=75  storage=Calibration  show_more=on  name_source=Use Parameter  data_type=int16  read_level=1  write_level=1  ovr_cals=on  view_as=Number  enum_struct={'Disabled', 'Enabled'}  vector_style=Wide Row  use_help_units=on  help='RPM rev limit for medium action to be taken'  units='RPM'  use_header_enum=off  row_header_enum={}  col_header_enum={}  use_min_max=on  min_val=0  max_val=inf  use_precision=off  precision=''  gain=1  offset=0  exp=1  use_mototune_group=on  mototune_group=motohawk_vardec_path(gcb)
  motohawk_calibration4 : MotoHawk_lib/Calibration & Probing Blocks/motohawk_calibration  nam='HardRevOffset'  val=100  storage=Calibration  show_more=on  name_source=Use Parameter  data_type=int16  read_level=1  write_level=1  ovr_cals=on  view_as=Number  enum_struct={'Disabled', 'Enabled'}  vector_style=Wide Row  use_help_units=on  help='RPM rev limit for hard action to be taken'  units='RPM'  use_header_enum=off  row_header_enum={}  col_header_enum={}  use_min_max=on  min_val=0  max_val=inf  use_precision=off  precision=''  gain=1  offset=0  exp=1  use_mototune_group=on  mototune_group=motohawk_vardec_path(gcb)
  Soft : Outport
  Medium : Outport  Port=2
  Hard : Outport  Port=3
  wires:
  Hysterisis2/1 -> Overspeed2/2
  Hysterisis1/1 -> Overspeed1/2
  Hysterisis/1 -> Overspeed/2
  motohawk_calibration1/1 -> Sum2/2, Sum1/2, Sum4/2
  motohawk_calibration/1 -> Sum2/1, Sum3/1, Sum5/1, Hysterisis/1
  RPM/1 -> Overspeed/1, Overspeed1/1, Overspeed2/1, Hysterisis/3, Hysterisis2/3, Hysterisis1/3
  motohawk_calibration2/1 -> Sum3/2
  Sum3/1 -> Sum1/1, Hysterisis1/1
  motohawk_calibration4/1 -> Sum5/2
  Sum5/1 -> Sum4/1, Hysterisis2/1
  Overspeed/1 -> Logical Operator3/1
  Logical Operator3/1 -> Soft/1
  Logical Operator4/1 -> Logical Operator3/2
  Overspeed1/1 -> Logical Operator4/1, Logical Operator5/1
  Logical Operator6/1 -> Logical Operator5/2
  Overspeed2/1 -> Logical Operator6/1, Hard/1
  Logical Operator5/1 -> Medium/1
  Sum2/1 -> Hysterisis/2
  Sum1/1 -> Hysterisis1/2
  Sum4/1 -> Hysterisis2/2

== system BaseEngineController_LS/Foreground/Control/VirtualSensors/AirCalcs/Capture Signal At Startup ==
  note: Count up to "BARO_Count" samples
  Signal_In : Inport
  Enable : EnablePort  StatesWhenEnabling=reset
  Add : Sum
  Add1 : Sum  Inputs=+-
  Collect Average : Subsystem  TreatAsAtomicUnit=on
  Constant : Constant  Value=int8(1)  SampleTime=-1
  Logical Operator : Logic  AllPortsSameDT=off  OutDataTypeStr=boolean
  Relational Operator : RelationalOperator  Operator=<=
  Relational Operator1 : RelationalOperator  Operator=>
  Sum : Sum  Inputs=++|  InputSameDT=on
  Switch : Switch  Threshold=1  ZeroCross=off  InputSameDT=on
  TwoSampleBuffer ToIgnore : Constant  Value=2  OutDataTypeStr=Inherit: Inherit via back propagation  SampleTime=-1
  Unit Delay : UnitDelay  SampleTime=-1
  motohawk_calibration : MotoHawk_lib/Calibration & Probing Blocks/motohawk_calibration  nam='BARO_Count'  val=int8(count)  storage=Calibration  show_more=on  name_source=Use Parameter  data_type=Inherit from 'Default Value'  read_level=1  write_level=1  ovr_cals=on  view_as=Number  enum_struct={'Disabled', 'Enabled'}  vector_style=Wide Row  use_help_units=on  help='Number of samples to average at key-up to produce signal value'  units=''  use_header_enum=off  row_header_enum={}  col_header_enum={}  use_min_max=off  min_val=-inf  max_val=inf  use_precision=off  precision=''  gain=1  offset=0  exp=1  use_mototune_group=on  mototune_group=motohawk_vardec_path(gcb)
  Signal_KeyUp : Outport
  wires:
  Sum/1 -> Switch/1, Relational Operator/1, Relational Operator1/1
  Relational Operator/1 -> Switch/2, Logical Operator/1
  Switch/1 -> Unit Delay/1, Add1/1
  Collect Average/1(Captured_Signal) -> Signal_KeyUp/1
  Signal_In/1 -> Collect Average/2(Signal)
  Unit Delay/1 -> Sum/1
  Constant/1 -> Sum/2
  motohawk_calibration/1 -> Add/1
  Add/1 -> Relational Operator/2, Switch/3
  TwoSampleBuffer ToIgnore/1 -> Add/2, Relational Operator1/2, Add1/2
  Logical Operator/1 -> Collect Average/Enable
  Relational Operator1/1 -> Logical Operator/2
  Add1/1 -> Collect Average/1(Count)

== system BaseEngineController_LS/Foreground/Control/VirtualSensors/AirCalcs/Running Baro Learn ==
  Eng State : Inport
  MAP : Inport  Port=2
  Compare To Constant : simulink/Logic and Bit Operations/Compare To Constant  SystemSampleTime=-1  relop=>  const=1  LogicOutDataTypeMode=uint8
  Data Type Conversion : DataTypeConversion  OutDataTypeStr=boolean
  Logical Operator : Logic  Inputs=3  AllPortsSameDT=off  OutDataTypeStr=boolean
  Product : Product  RndMeth=Zero
  Relational Operator : RelationalOperator  OutDataTypeStr=boolean
  Relational Operator1 : RelationalOperator  OutDataTypeStr=boolean
  Relational Operator2 : RelationalOperator  OutDataTypeStr=boolean
  Time Since Enabled (With Input)1 : motohawk_control_primitives_lib/Time Since Enabled (With Input)1  SystemSampleTime=-1  nam='BaroLearnTmr'  samp_time=-1  init=0  upperlim=16000
  motohawk_calibration : MotoHawk_lib/Calibration & Probing Blocks/motohawk_calibration  nam='BaroLearn_Tm'  val=.2  storage=Calibration  show_more=on  name_source=Use Parameter  data_type=Inherit from 'Default Value'  read_level=1  write_level=1  ovr_cals=on  view_as=Number  enum_struct={'Disabled', 'Enabled'}  vector_style=Wide Row  use_help_units=on  help=''  units='sec'  use_header_enum=off  row_header_enum={}  col_header_enum={}  use_min_max=on  min_val=0  max_val=100  use_precision=off  precision=''  gain=1  offset=0  exp=1  use_mototune_group=off  mototune_group=motohawk_vardec_path(gcb)
  motohawk_calibration1 : MotoHawk_lib/Calibration & Probing Blocks/motohawk_calibration  nam='BaroLearn_TPSPos'  val=95  storage=Calibration  show_more=on  name_source=Use Parameter  data_type=Inherit from 'Default Value'  read_level=1  write_level=1  ovr_cals=on  view_as=Number  enum_struct={'Disabled', 'Enabled'}  vector_style=Wide Row  use_help_units=on  help=''  units='%'  use_header_enum=off  row_header_enum={}  col_header_enum={}  use_min_max=on  min_val=0  max_val=100  use_precision=off  precision=''  gain=1  offset=0  exp=1  use_mototune_group=off  mototune_group=motohawk_vardec_path(gcb)
  motohawk_calibration2 : MotoHawk_lib/Calibration & Probing Blocks/motohawk_calibration  nam='BaroLearn_MAP'  val=95  storage=Calibration  show_more=on  name_source=Use Parameter  data_type=Inherit from 'Default Value'  read_level=1  write_level=1  ovr_cals=on  view_as=Number  enum_struct={'Disabled', 'Enabled'}  vector_style=Wide Row  use_help_units=on  help=''  units='kPa'  use_header_enum=off  row_header_enum={}  col_header_enum={}  use_min_max=on  min_val=0  max_val=100  use_precision=off  precision=''  gain=1  offset=0  exp=1  use_mototune_group=off  mototune_group=motohawk_vardec_path(gcb)
  motohawk_data_read : MotoHawk_lib/Data Storage Blocks/motohawk_data_read  source=Lookup By Name  structure=Scalar  operation=Read scalar from location by index  sz_vec=4  sz_row=2  sz_col=3  typ=double  nam='TPSFinal'  checkNull=on  struct_inst_name='MyData'  struct_nam='MyStruct'
  Enbl : Outport  OutDataTypeStr=boolean
  wires:
  motohawk_data_read/1 -> Relational Operator/1
  motohawk_calibration1/1 -> Relational Operator/2
  MAP/1 -> Relational Operator1/1
  motohawk_calibration2/1 -> Relational Operator1/2
  Relational Operator/1 -> Logical Operator/1
  Relational Operator1/1 -> Logical Operator/2
  Eng State/1 -> Compare To Constant/1
  Compare To Constant/1 -> Logical Operator/3
  Logical Operator/1 -> Time Since Enabled (With Input)1/1, Product/1
  Time Since Enabled (With Input)1/1 -> Relational Operator2/1
  motohawk_calibration/1 -> Relational Operator2/2
  Relational Operator2/1 -> Product/2
  Product/1 -> Data Type Conversion/1
  Data Type Conversion/1 -> Enbl/1
